simulink model "rotational_system_sim_extra"  (R2013a)
settings: Solver=ode45  StartTime=0.0  StopTime=10  RelTol=1e-3
values from neighbouring files (symbols this model uses):
  b = 0.002    [rocket_roll_validation.m]    (also in rocket_roll_validation_excess_code_not_pretty.m; rotational_system.m; trail.m = 0.02)
  ct = 0.2    [rocket_roll_validation.m]    (also in rocket_roll_validation_excess_code_not_pretty.m; rotational_system.m = 0.1)
  fr = 2.75*.0254    (= 0.06985)    [rocket_roll_validation.m]    (also in rocket_roll_validation_excess_code_not_pretty.m; rotational_system.m; trail.m)
  Ftot = 11    [rocket_roll_validation.m]    (also in rocket_roll_validation_excess_code_not_pretty.m; rotational_system.m = 5.5)
  hz = 10    [rocket_roll_validation.m]    (also in rocket_roll_validation_excess_code_not_pretty.m; rotational_system.m)
  I = 0.0198    [rocket_roll_validation.m]    (also in rocket_roll_validation_excess_code_not_pretty.m; rotational_system.m; trail.m = 0.0197946818182)
  Tau = 0.02    [rocket_roll_validation.m]    (also in rocket_roll_validation_excess_code_not_pretty.m; rotational_system.m = 0.009)
libraries: simulink x4
settings Model: Creator=karnell  LastModifiedBy=kenny
settings DataIOCC: SignalLoggingSaveFormat=ModelDataLogs
settings DebuggingCC: MultiTaskDSMMsg=warning  MultiTaskCondExecSysMsg=none  StateNameClashWarn=none  StrictBusMsg=None
settings RTWCC: IncludeERTFirstTime=on

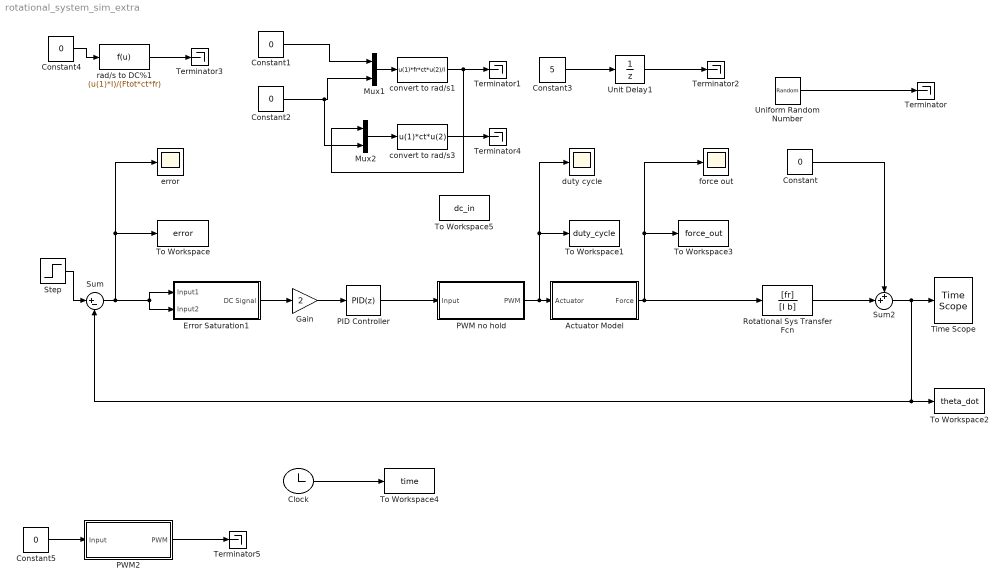
== system rotational_system_sim_extra ==
  Actuator Model : Subsystem
  Clock : Clock
  Constant{,1..2,4..5} (5 alike) : Constant  Value=0
  Constant3 : Constant  Value=5
  Error Saturation1 : Subsystem
  Gain : Gain  Gain=2
  Mux1 : Mux  Inputs=2
  Mux2 : Mux  Inputs=2
  PID Controller : simulink/Continuous/PID Controller  Controller=PID  TimeDomain=Discrete-time  SampleTime=.003  IntegratorMethod=Forward Euler  FilterMethod=Forward Euler  Form=Parallel  P=.2  I=0  D=0  N=100  InitialConditionSource=internal  InitialConditionForIntegrator=0  InitialConditionForFilter=0  ExternalReset=none  LimitOutput=off  UpperSaturationLimit=inf  LowerSaturationLimit=-inf  LinearizeAsGain=on  AntiWindupMode=none  Kb=1  TrackingMode=off  Kt=1  PParamMin=[]  PParamMax=[]  IParamMin=[]  IParamMax=[]  DParamMin=[]  DParamMax=[]  NParamMin=[]  NParamMax=[]  KbParamMin=[]  KbParamMax=[]  KtParamMin=[]  KtParamMax=[]  POutMin=[]  POutMax=[]  IOutMin=[]  IOutMax=[]  DOutMin=[]  DOutMax=[]  NOutMin=[]  NOutMax=[]  KbOutMin=[]  KbOutMax=[]  KtOutMin=[]  KtOutMax=[]  IntegratorOutMin=[]  IntegratorOutMax=[]  FilterOutMin=[]  FilterOutMax=[]  SumOutMin=[]  SumOutMax=[]  SumI1OutMin=[]  SumI1OutMax=[]  SumI2OutMin=[]  SumI2OutMax=[]  SumI3OutMin=[]  SumI3OutMax=[]  SumDOutMin=[]  SumDOutMax=[]  SaturationOutMin=[]  SaturationOutMax=[]  IntegratorContinuousStateAttributes=''  IntegratorStateMustResolveToSignalObject=off  IntegratorRTWStateStorageClass=Auto  FilterContinuousStateAttributes=''  FilterStateMustResolveToSignalObject=off  FilterRTWStateStorageClass=Auto
  PWM no hold : Subsystem
  PWM2 : Subsystem
  Rotational Sys Transfer Fcn : TransferFcn  Numerator=[fr]  Denominator=[I b]
  Step : Step  Time=0  After=1.03  SampleTime=0
  Sum : Sum  Inputs=|+-
  Sum2 : Sum  Inputs=++|
  Terminator{,1..5} (6 alike) : Terminator
  Time Scope : TimeScope  DefaultConfigurationName=spbscopes.TimeScopeBlockCfg
      settings: CopyFcn=scopeextensions.ScopeBlock.callback(gcbh, 'onBlockCopy', gcbh);  DeleteFcn=scopeextensions.ScopeBlock.callback(gcbh, 'onBlockDelete');  PreSaveFcn=scopeextensions.ScopeBlock.callback(gcbh, 'onModelSave');  NameChangeFcn=scopeextensions.ScopeBlock.callback(gcbh, 'onBlockRename');  CloseFcn=scopeextensions.ScopeBlock.callback(gcbh, 'onBlockClose');  PreDeleteFcn=scopeextensions.ScopeBlock.callback(gcbh, 'onBlockPreDelete');
  To Workspace : ToWorkspace  VariableName=error  SampleTime=-1  SaveFormat=Structure With Time
  To Workspace1 : ToWorkspace  VariableName=duty_cycle  SampleTime=-1  SaveFormat=Structure With Time
  To Workspace2 : ToWorkspace  VariableName=theta_dot  SampleTime=-1  SaveFormat=Structure With Time
  To Workspace3 : ToWorkspace  VariableName=force_out  SampleTime=-1
  To Workspace4 : ToWorkspace  VariableName=time  SampleTime=-1
  To Workspace5 : ToWorkspace  VariableName=dc_in  SampleTime=-1  SaveFormat=Structure With Time
  Uniform Random Number : UniformRandomNumber  Minimum=-.09  Maximum=.09  SampleTime=0.1
  Unit Delay1 : UnitDelay  SampleTime=-1
  convert to rad/s1 : Fcn  Expr=u(1)*fr*ct*u(2)/I
  convert to rad/s3 : Fcn  Expr=u(1)*ct*u(2)
  duty cycle : Scope
      settings: YMin=-1  YMax=2
  error : Scope
      settings: SaveName=ScopeData2
  force out : Scope
  rad/s to DC%1 : Fcn  Expr=(u(1)*I)/(Ftot*ct*fr)
  wires:
  Sum/1 -> Error Saturation1/2(Input2), Error Saturation1/1(Input1), error/1, To Workspace/1
  PWM no hold/1(PWM) -> Actuator Model/1(Actuator), duty cycle/1, To Workspace1/1
  Gain/1 -> PID Controller/1
  Step/1 -> Sum/1
  Clock/1 -> To Workspace4/1
  Sum2/1 -> Time Scope/1, Sum/2, To Workspace2/1
  Rotational Sys Transfer Fcn/1 -> Sum2/2
  convert to rad/s1/1 -> Mux2/1, Terminator1/1
  Constant1/1 -> Mux1/1
  Constant2/1 -> Mux2/2, Mux1/2
  Mux1/1 -> convert to rad/s1/1
  Constant/1 -> Sum2/1
  Uniform Random Number/1 -> Terminator/1
  Mux2/1 -> convert to rad/s3/1
  Constant3/1 -> Unit Delay1/1
  Constant4/1 -> rad/s to DC%1/1
  rad/s to DC%1/1 -> Terminator3/1
  Unit Delay1/1 -> Terminator2/1
  convert to rad/s3/1 -> Terminator4/1
  Actuator Model/1(Force) -> Rotational Sys Transfer Fcn/1, force out/1, To Workspace3/1
  Error Saturation1/1(DC Signal) -> Gain/1
  PID Controller/1 -> PWM no hold/1(Input)
  Constant5/1 -> PWM2/1(Input)
  PWM2/1(PWM) -> Terminator5/1

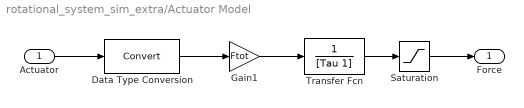
== system rotational_system_sim_extra/Actuator Model ==
  Actuator : Inport
  Data Type Conversion : DataTypeConversion
  Gain1 : Gain  Gain=Ftot
  Saturation : Saturate  UpperLimit=Ftot  LowerLimit=-Ftot
  Transfer Fcn : TransferFcn  Denominator=[Tau 1]
  Force : Outport
  wires:
  Actuator/1 -> Data Type Conversion/1
  Transfer Fcn/1 -> Saturation/1
  Data Type Conversion/1 -> Gain1/1
  Saturation/1 -> Force/1
  Gain1/1 -> Transfer Fcn/1

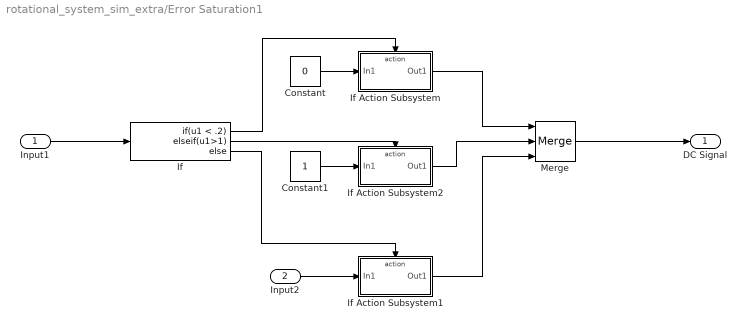
== system rotational_system_sim_extra/Error Saturation1 ==
  Input1 : Inport
  Input2 : Inport  Port=2
  Constant : Constant  Value=0
  Constant1 : Constant
  If : If  IfExpression=u1 < .2  ElseIfExpressions=u1>1
  If Action Subsystem : Subsystem  TreatAsAtomicUnit=on
  If Action Subsystem1 : Subsystem  TreatAsAtomicUnit=on
  If Action Subsystem2 : Subsystem  TreatAsAtomicUnit=on
  Merge : Merge  Inputs=3
  DC Signal : Outport
  wires:
  Input1/1 -> If/1
  Merge/1 -> DC Signal/1
  If Action Subsystem/1(Out1) -> Merge/1
  Constant/1 -> If Action Subsystem/1(In1)
  If/1 -> If Action Subsystem/Action
  If/3 -> If Action Subsystem1/Action
  If Action Subsystem1/1(Out1) -> Merge/3
  Input2/1 -> If Action Subsystem1/1(In1)
  If/2 -> If Action Subsystem2/Action
  If Action Subsystem2/1(Out1) -> Merge/2
  Constant1/1 -> If Action Subsystem2/1(In1)

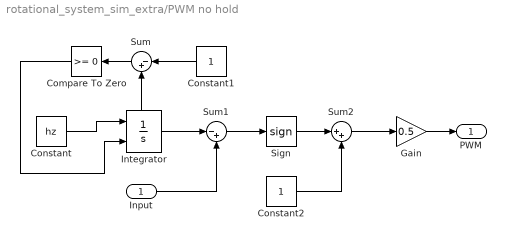
== system rotational_system_sim_extra/PWM no hold ==
  Input : Inport
  Compare To Zero : simulink/Logic and Bit Operations/Compare To Zero  relop=>=  OutDataTypeStr=boolean
  Constant : Constant  Value=hz
  Constant1 : Constant
  Constant2 : Constant
  Gain : Gain  Gain=0.5
  Integrator : Integrator  ExternalReset=rising  ShowStatePort=on
  Sign : Signum
  Sum : Sum  Inputs=|-+
  Sum1 : Sum  Inputs=|-+
  Sum2 : Sum  Inputs=|++
  PWM : Outport
  wires:
  Constant1/1 -> Sum/1
  Sum/1 -> Compare To Zero/1
  Integrator/1 -> Sum1/1
  Input/1 -> Sum1/2
  Sum1/1 -> Sign/1
  Sign/1 -> Sum2/1
  Constant2/1 -> Sum2/2
  Sum2/1 -> Gain/1
  Gain/1 -> PWM/1
  Constant/1 -> Integrator/1
  Compare To Zero/1 -> Integrator/2
  Integrator/State -> Sum/2

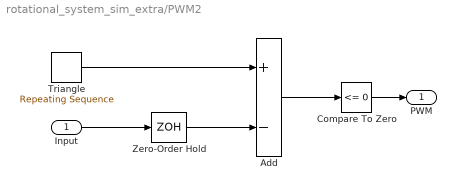
== system rotational_system_sim_extra/PWM2 ==
  Input : Inport
  Add : Sum  Inputs=+-  SampleTime=1/10
  Compare To Zero : simulink/Logic and Bit Operations/Compare To Zero  relop=<=  OutDataTypeStr=uint8
  Triangle : simulink/Sources/Repeating Sequence  rep_seq_t=[0 1/hz/4 3/hz/4 1/hz]  rep_seq_y=[0.5 0 1 0.5]
  Zero-Order Hold : ZeroOrderHold  SampleTime=1/10
  PWM : Outport
  wires:
  Zero-Order Hold/1 -> Add/2
  Compare To Zero/1 -> PWM/1
  Add/1 -> Compare To Zero/1
  Input/1 -> Zero-Order Hold/1
  Triangle/1 -> Add/1

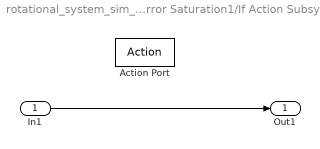
== system rotational_system_sim_extra/Error Saturation1/If Action Subsystem ==
  In1 : Inport
  Action Port : ActionPort  ActionType=then
  Out1 : Outport
  wires:
  In1/1 -> Out1/1

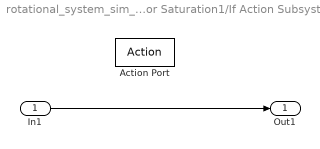
== system rotational_system_sim_extra/Error Saturation1/If Action Subsystem1 ==
  In1 : Inport
  Action Port : ActionPort  ActionType=else
  Out1 : Outport
  wires:
  In1/1 -> Out1/1

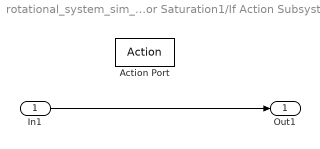
== system rotational_system_sim_extra/Error Saturation1/If Action Subsystem2 ==
  In1 : Inport
  Action Port : ActionPort  ActionType=elseif
  Out1 : Outport
  wires:
  In1/1 -> Out1/1
